simulink model "DconstZ_snt"  (R2025b)
settings: Solver=ode45  StartTime=0.0  StopTime=10.0  RelTol=1e-3  EnableMultiTasking=on
undefined symbols (not defined in the file or in its folder): L65_PA, L65_PB, L65_PC, L65_QA, L65_QB, L65_QC
libraries: fl_lib x12
settings Model: Creator=gdudgeon  LastModifiedBy=gdudgeon
settings SolverCC: AlgebraicLoopSolver=TrustRegion
settings DataIOCC: LimitDataPoints=on  SaveFormat=Array  ReturnWorkspaceOutputs=off
settings OptimizationCC: ExpressionDepthLimit=2147483647.0  LifeSpan=inf
settings DebuggingCC: UnderspecifiedInitializationDetection=Classic  MergeDetectMultiDrivingBlocksExec=none  SolverPrmCheckMsg=warning  UnconnectedInputMsg=warning  UnconnectedOutputMsg=warning  UnconnectedLineMsg=warning  StateNameClashWarn=warning  SFUnexpectedBacktrackingDiag=warning  SFNoUnconditionalDefaultTransitionDiag=warning  SFExecutionAtInitializationDiag=none  ArithmeticOperatorsInVariantConditions=warning
settings HardwareCC: ProdBitPerPointer=32.0  ProdBitPerSizeT=32.0  ProdBitPerPtrDiffT=32.0  ProdLargestAtomicFloat=None  ProdIntDivRoundTo=Undefined  ProdEndianess=Unspecified  ProdWordSize=32.0  ProdHWDeviceType=32-bit Generic
settings ModelReferenceCC: EnableRefExpFcnMdlSchedulingChecks=on  PropagateSignalLabelsOutOfModel=off
settings SFSimCC: SimUseLocalCustomCode=off  CustomCodeUndefinedFunction=UseInterfaceOnly
settings RTWCC: RTWUseLocalCustomCode=off  GPUComputeCapability=3.5
settings CodeAppCC: StateflowObjectComments=on
settings GRTTargetCC: TargetLangStandard=C89/C90 (ANSI)
settings ConfigComp: CovMetricSettings=dw  CovSaveCumulativeToWorkspaceVar=on  CovSaveSingleToWorkspaceVar=on  CovExternalEMLEnable=off
settings SimscapeCC: SimscapeNormalizeSystem=off

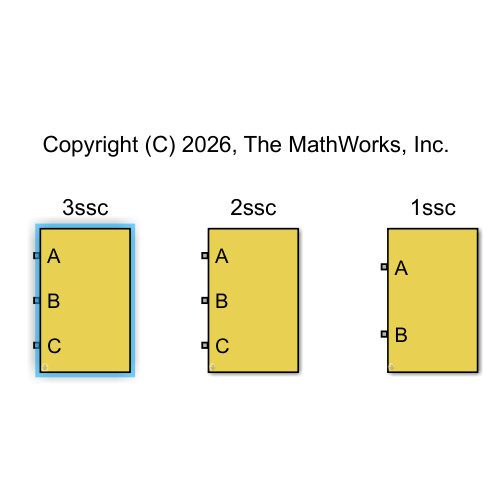
[thumbnail: Simulink's stored preview of the top-level diagram]
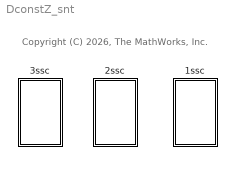
== system DconstZ_snt ==
  note: Copyright (C) 2026, The MathWorks, Inc.
  1ssc : Subsystem  mask{t1=t, PA1=L65_PA, QA1=L65_QA, PB1=L65_PB, QB1=L65_QB, PC1=L65_PC, QC1=L65_QC}
      mask prompts: t1 "Time (s)"; PA1 "PA (W)"; QA1 "QA (VAr)"; PB1 "PB (W)"; QB1 "QB (VAr)"; PC1 "PC (W)"; QC1 "QC (VAr)"
  2ssc : Subsystem  mask{t1=t, PA1=L65_PA, QA1=L65_QA, PB1=L65_PB, QB1=L65_QB, PC1=L65_PC, QC1=L65_QC}
      mask prompts: t1 "Time (s)"; PA1 "PA (W)"; QA1 "QA (VAr)"; PB1 "PB (W)"; QB1 "QB (VAr)"; PC1 "PC (W)"; QC1 "QC (VAr)"
  3ssc : Subsystem  mask{t1=t, PA1=L65_PA, QA1=L65_QA, PB1=L65_PB, QB1=L65_QB, PC1=L65_PC, QC1=L65_QC}
      mask prompts: t1 "Time (s)"; PA1 "PA (W)"; QA1 "QA (VAr)"; PB1 "PB (W)"; QB1 "QB (VAr)"; PC1 "PC (W)"; QC1 "QC (VAr)"

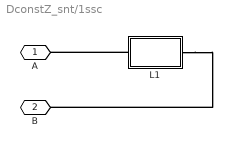
== system DconstZ_snt/1ssc ==
  L1 : Subsystem  mask{Vrms=4.16e3, f=60, P=PA1(1), Q=QA1(1)}
      mask prompts: Vrms "Vrms (V)"; f "freq (Hz)"; P "P (W)"; Q "Q (VA)"
      mask init:
      | % R = Vrms^2/P/(1+Q^2/P^2);
      | % 
      | % L = R*Q/(2*pi*f)/P;
      | 
      | R = (Vrms^2)/P;
      | 
      | L = (Vrms^2)/(2*pi*f)/Q;
  A : PMIOPort  Side=Left
  B : PMIOPort  Port=2  Side=Left
  connections:
  L1/RConn1 -- B/RConn1
  L1/LConn1 -- A/RConn1

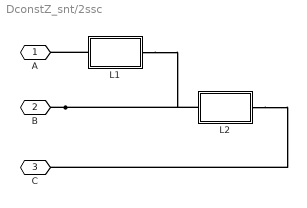
== system DconstZ_snt/2ssc ==
  L1 : Subsystem  mask{Vrms=4.16e3, f=60, P=PA1(1), Q=QA1(1)}
      mask prompts: Vrms "Vrms (V)"; f "freq (Hz)"; P "P (W)"; Q "Q (VA)"
      mask init:
      | % R = Vrms^2/P/(1+Q^2/P^2);
      | % 
      | % L = R*Q/(2*pi*f)/P;
      | 
      | R = (Vrms^2)/P;
      | 
      | L = (Vrms^2)/(2*pi*f)/Q;
  L2 : Subsystem  mask{Vrms=4.16e3, f=60, P=PB1(1), Q=QB1(1)}
      mask prompts: Vrms "Vrms (V)"; f "freq (Hz)"; P "P (W)"; Q "Q (VA)"
      mask init:
      | % R = Vrms^2/P/(1+Q^2/P^2);
      | % 
      | % L = R*Q/(2*pi*f)/P;
      | 
      | R = (Vrms^2)/P;
      | 
      | L = (Vrms^2)/(2*pi*f)/Q;
  A : PMIOPort  Side=Left
  B : PMIOPort  Port=2  Side=Left
  C : PMIOPort  Port=3  Side=Left
  connections:
  L1/LConn1 -- A/RConn1
  B/RConn1 -- L2/LConn1 -- L1/RConn1
  L2/RConn1 -- C/RConn1

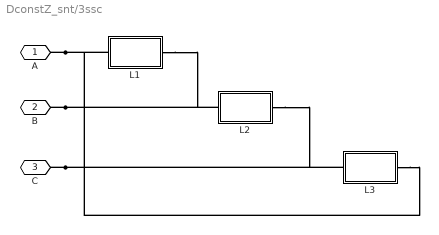
== system DconstZ_snt/3ssc ==
  L1 : Subsystem  mask{Vrms=4.16e3, f=60, P=PA1(1), Q=QA1(1)}
      mask prompts: Vrms "Vrms (V)"; f "freq (Hz)"; P "P (W)"; Q "Q (VA)"
      mask init:
      | % R = Vrms^2/P/(1+Q^2/P^2);
      | % 
      | % L = R*Q/(2*pi*f)/P;
      | 
      | R = (Vrms^2)/P;
      | 
      | L = (Vrms^2)/(2*pi*f)/Q;
  L2 : Subsystem  mask{Vrms=4.16e3, f=60, P=PB1(1), Q=QB1(1)}
      mask prompts: Vrms "Vrms (V)"; f "freq (Hz)"; P "P (W)"; Q "Q (VA)"
      mask init:
      | % R = Vrms^2/P/(1+Q^2/P^2);
      | % 
      | % L = R*Q/(2*pi*f)/P;
      | 
      | R = (Vrms^2)/P;
      | 
      | L = (Vrms^2)/(2*pi*f)/Q;
  L3 : Subsystem  mask{Vrms=4.16e3, f=60, P=PC1(1), Q=QC1(1)}
      mask prompts: Vrms "Vrms (V)"; f "freq (Hz)"; P "P (W)"; Q "Q (VA)"
      mask init:
      | % R = Vrms^2/P/(1+Q^2/P^2);
      | % 
      | % L = R*Q/(2*pi*f)/P;
      | 
      | R = (Vrms^2)/P;
      | 
      | L = (Vrms^2)/(2*pi*f)/Q;
  A : PMIOPort  Side=Left
  B : PMIOPort  Port=2  Side=Left
  C : PMIOPort  Port=3  Side=Left
  connections:
  C/RConn1 -- L3/LConn1 -- L2/RConn1
  B/RConn1 -- L1/RConn1 -- L2/LConn1
  A/RConn1 -- L3/RConn1 -- L1/LConn1

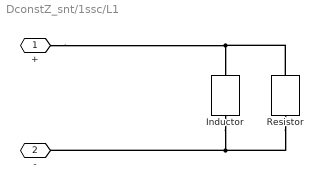
== system DconstZ_snt/1ssc/L1 ==
  Inductor : fl_lib/Electrical/Electrical Elements/Inductor  l=L H  r=0 Ohm  g=0 1/Ohm  i_specify=off  i_priority=None  i=0 A  i_nominal_specify=off  i_nominal_value=1  i_nominal_unit=A  v_specify=off  v_priority=None  v=0 V  v_nominal_specify=off  v_nominal_value=1  v_nominal_unit=V  i_L_specify=off  i_L_priority=High  i_L=0 A  i_L_nominal_specify=off  i_L_nominal_value=1  i_L_nominal_unit=A
  Resistor : fl_lib/Electrical/Electrical Elements/Resistor  R=R Ohm  i_specify=on  i_priority=Low  i=0 A  i_nominal_specify=off  i_nominal_value=1  i_nominal_unit=A  v_specify=on  v_priority=Low  v=0 V  v_nominal_specify=off  v_nominal_value=1  v_nominal_unit=V
  " +" : PMIOPort  Side=Left
  - : PMIOPort  Port=2  Side=Right
  connections:
  Resistor/RConn1 -- Inductor/RConn1 -- -/RConn1
  " +"/RConn1 -- Inductor/LConn1 -- Resistor/LConn1

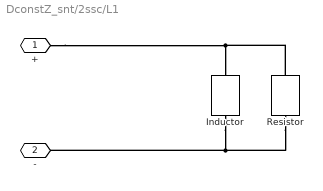
== system DconstZ_snt/2ssc/L1 ==
  Inductor : fl_lib/Electrical/Electrical Elements/Inductor  l=L H  r=0 Ohm  g=0 1/Ohm  i_specify=on  i_priority=Low  i=0 A  i_nominal_specify=off  i_nominal_value=1  i_nominal_unit=A  v_specify=on  v_priority=Low  v=0 V  v_nominal_specify=off  v_nominal_value=1  v_nominal_unit=V  i_L_specify=on  i_L_priority=Low  i_L=0 A  i_L_nominal_specify=off  i_L_nominal_value=1  i_L_nominal_unit=A
  Resistor : fl_lib/Electrical/Electrical Elements/Resistor  R=R Ohm  i_specify=on  i_priority=Low  i=0 A  i_nominal_specify=off  i_nominal_value=1  i_nominal_unit=A  v_specify=on  v_priority=Low  v=0 V  v_nominal_specify=off  v_nominal_value=1  v_nominal_unit=V
  " +" : PMIOPort  Side=Left
  - : PMIOPort  Port=2  Side=Right
  connections:
  Resistor/RConn1 -- Inductor/RConn1 -- -/RConn1
  " +"/RConn1 -- Inductor/LConn1 -- Resistor/LConn1

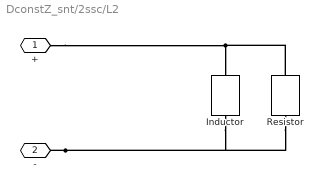
== system DconstZ_snt/2ssc/L2 ==
  Inductor : fl_lib/Electrical/Electrical Elements/Inductor  l=L H  r=0 Ohm  g=0 1/Ohm  i_specify=on  i_priority=Low  i=0 A  i_nominal_specify=off  i_nominal_value=1  i_nominal_unit=A  v_specify=on  v_priority=Low  v=0 V  v_nominal_specify=off  v_nominal_value=1  v_nominal_unit=V  i_L_specify=on  i_L_priority=Low  i_L=0 A  i_L_nominal_specify=off  i_L_nominal_value=1  i_L_nominal_unit=A
  Resistor : fl_lib/Electrical/Electrical Elements/Resistor  R=R Ohm  i_specify=on  i_priority=Low  i=0 A  i_nominal_specify=off  i_nominal_value=1  i_nominal_unit=A  v_specify=on  v_priority=Low  v=0 V  v_nominal_specify=off  v_nominal_value=1  v_nominal_unit=V
  " +" : PMIOPort  Side=Left
  - : PMIOPort  Port=2  Side=Right
  connections:
  Resistor/LConn1 -- Inductor/LConn1 -- " +"/RConn1
  -/RConn1 -- Inductor/RConn1 -- Resistor/RConn1

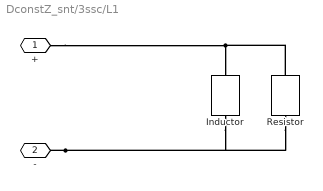
== system DconstZ_snt/3ssc/L1 ==
  Inductor : fl_lib/Electrical/Electrical Elements/Inductor  l=L H  r=0 Ohm  g=0 1/Ohm  i_specify=on  i_priority=Low  i=0 A  i_nominal_specify=off  i_nominal_value=1  i_nominal_unit=A  v_specify=on  v_priority=Low  v=0 V  v_nominal_specify=off  v_nominal_value=1  v_nominal_unit=V  i_L_specify=on  i_L_priority=Low  i_L=0 A  i_L_nominal_specify=off  i_L_nominal_value=1  i_L_nominal_unit=A
  Resistor : fl_lib/Electrical/Electrical Elements/Resistor  R=R Ohm  i_specify=on  i_priority=Low  i=0 A  i_nominal_specify=off  i_nominal_value=1  i_nominal_unit=A  v_specify=on  v_priority=Low  v=0 V  v_nominal_specify=off  v_nominal_value=1  v_nominal_unit=V
  " +" : PMIOPort  Side=Left
  - : PMIOPort  Port=2  Side=Right
  connections:
  Resistor/LConn1 -- Inductor/LConn1 -- " +"/RConn1
  -/RConn1 -- Inductor/RConn1 -- Resistor/RConn1

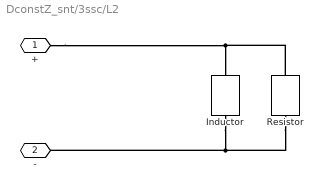
== system DconstZ_snt/3ssc/L2 ==
  Inductor : fl_lib/Electrical/Electrical Elements/Inductor  l=L H  r=0 Ohm  g=0 1/Ohm  i_specify=on  i_priority=Low  i=0 A  i_nominal_specify=off  i_nominal_value=1  i_nominal_unit=A  v_specify=on  v_priority=Low  v=0 V  v_nominal_specify=off  v_nominal_value=1  v_nominal_unit=V  i_L_specify=on  i_L_priority=Low  i_L=0 A  i_L_nominal_specify=off  i_L_nominal_value=1  i_L_nominal_unit=A
  Resistor : fl_lib/Electrical/Electrical Elements/Resistor  R=R Ohm  i_specify=on  i_priority=Low  i=0 A  i_nominal_specify=off  i_nominal_value=1  i_nominal_unit=A  v_specify=on  v_priority=Low  v=0 V  v_nominal_specify=off  v_nominal_value=1  v_nominal_unit=V
  " +" : PMIOPort  Side=Left
  - : PMIOPort  Port=2  Side=Right
  connections:
  Resistor/RConn1 -- Inductor/RConn1 -- -/RConn1
  " +"/RConn1 -- Inductor/LConn1 -- Resistor/LConn1

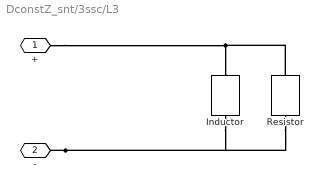
== system DconstZ_snt/3ssc/L3 ==
  Inductor : fl_lib/Electrical/Electrical Elements/Inductor  l=L H  r=0 Ohm  g=0 1/Ohm  i_specify=on  i_priority=Low  i=0 A  i_nominal_specify=off  i_nominal_value=1  i_nominal_unit=A  v_specify=on  v_priority=Low  v=0 V  v_nominal_specify=off  v_nominal_value=1  v_nominal_unit=V  i_L_specify=on  i_L_priority=Low  i_L=0 A  i_L_nominal_specify=off  i_L_nominal_value=1  i_L_nominal_unit=A
  Resistor : fl_lib/Electrical/Electrical Elements/Resistor  R=R Ohm  i_specify=on  i_priority=Low  i=0 A  i_nominal_specify=off  i_nominal_value=1  i_nominal_unit=A  v_specify=on  v_priority=Low  v=0 V  v_nominal_specify=off  v_nominal_value=1  v_nominal_unit=V
  " +" : PMIOPort  Side=Left
  - : PMIOPort  Port=2  Side=Right
  connections:
  Resistor/LConn1 -- Inductor/LConn1 -- " +"/RConn1
  -/RConn1 -- Inductor/RConn1 -- Resistor/RConn1
